simulink model "Demo1_P1C2"  (R2025b)
settings: Solver=VariableStepAuto  StartTime=0.0  StopTime=3  RelTol=1e-3
settings Model: Creator=abadirwahba  LastModifiedBy=abadirwahba

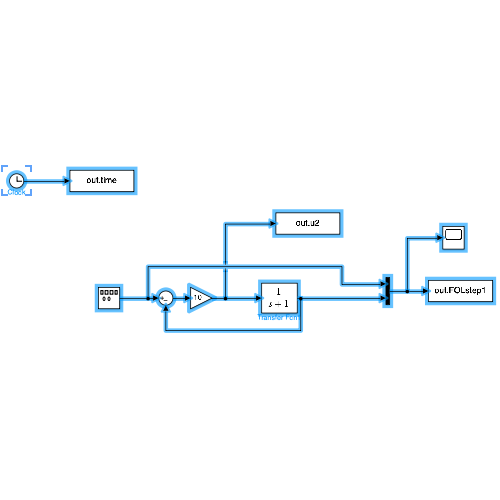
[thumbnail: Simulink's stored preview of the top-level diagram]
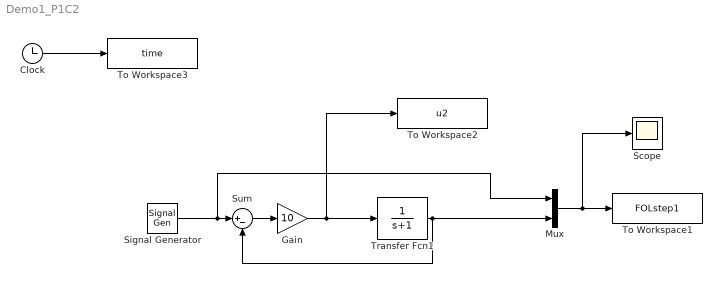
== system Demo1_P1C2 ==
  Clock : Clock
  Gain : Gain  Gain=10
  Mux : Mux  Inputs=2
  Scope : Scope
      settings: ActiveDisplayYMinimum=-1.25  ActiveDisplayYMaximum=1.25
  Signal Generator : SignalGenerator  WaveForm=square  Frequency=0.5
  Sum : Sum  Inputs=|+-
  To Workspace1 : ToWorkspace  VariableName=FOLstep1  SampleTime=-1
  To Workspace2 : ToWorkspace  VariableName=u2  SampleTime=-1
  To Workspace3 : ToWorkspace  VariableName=time  SampleTime=-1
  Transfer Fcn1 : TransferFcn  Denominator=[1 1]
  wires:
  Transfer Fcn1/1 -> Sum/2, Mux/2
  Signal Generator/1 -> Sum/1, Mux/1
  Mux/1 -> Scope/1, To Workspace1/1
  Sum/1 -> Gain/1
  Gain/1 -> To Workspace2/1, Transfer Fcn1/1
  Clock/1 -> To Workspace3/1
